simulink library "TireBody_Parameterized"  (R2026a)
settings: Solver=VariableStepAuto
undefined symbols (not defined in the file): X, Y, Z
libraries: sm_lib x4
Description:
  | Copyright 2020-2026 The MathWorks, Inc.
settings Model: Creator=smiller  LastModifiedBy=smiller

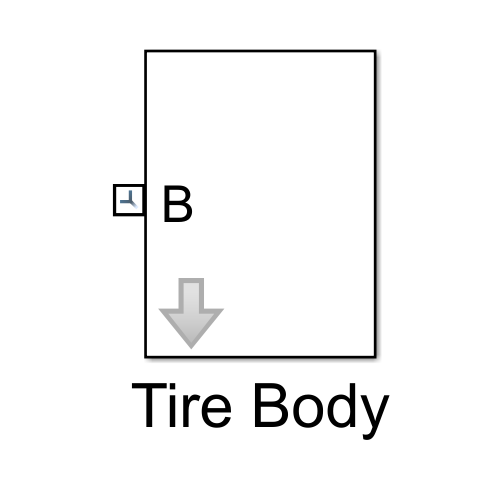
[thumbnail: Simulink's stored preview of the top-level diagram]
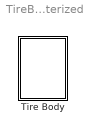
== system TireBody_Parameterized ==
  Tire Body : Subsystem  mask(Parameterized Tire Solid){radius=0.4225, rim_radius=0.3048, width=0.235, rim_width=0.235*0.1, mass=10, rim_mass=0, tire_inertia=[1 2], rim_inertia=[0 0], popup_leftRight=Left, clr_tyre=[0.5 0.5 0.5], opc_tyre=1.0, clr_rim=[0.8 0.8 0.8], opc_rim=0.5}
      mask prompts: popup_leftRight "Left/Right"
      mask help: Model mass, inertia and geometry of tire and rim.
      mask init:
      | % Change rim location if wheel is on right side
      | if (popup_leftRight == 1)
      |     rhs_tire = 1;
      | elseif(popup_leftRight == 2)
      |     rhs_tire = -1;
      | end
      | 
      | Imat = [tire_inertia(1)+rim_inertia(1) 0 0; 0 tire_inertia(1)+rim_inertia(1) 0; 0 0 tire_inertia(2)+rim_inertia(2)];
      mask TypeOptions popup_leftRight: Left | Right
      mask TypeOptions clr_tyre: Tire/GraphicDiffuseColor
      mask TypeOptions opc_tyre: Tire/GraphicOpacity
      mask TypeOptions clr_rim: Rim/GraphicDiffuseColor
      mask TypeOptions opc_rim: Rim/GraphicOpacity
      mask DialogControl cont_tyre Prompt: Tire Geometry
      mask DialogControl group_tyre_dim Prompt: Dimensions
      mask DialogControl text_tyre_tire Prompt: Tyre
      mask DialogControl text_tyre_rim Prompt: Rim
      mask DialogControl text_tyre_dim_radius Prompt: Radius (m)
      mask DialogControl text_tyre_dim_width Prompt: Width (m)
      mask DialogControl text_tyre_mass Prompt: Mass (kg)
      mask DialogControl text_tyre_inertia Prompt: Inertia [Ixx Iyy]
      mask DialogControl cont_tyre_vis Prompt: Visualization
      mask DialogControl text_vis_tyre_clr Prompt: Color [RGB]
      mask DialogControl text_vis_tyre_opc Prompt: Opacity (0-1)
      mask DialogControl text_vis_tyre_tyre Prompt: Tyre
      mask DialogControl text_vis_tyre_rim Prompt: Rim

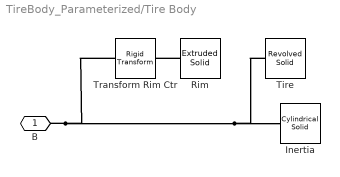
== system TireBody_Parameterized/Tire Body ==
  Inertia : sm_lib/Body Elements/Cylindrical Solid  CylinderRadius=0.001  CylinderRadiusUnits=m  CylinderLength=0.001  CylinderLengthUnits=m  ExportEntireGeometry=off  InertiaType=Custom  BasedOnType=Density  Density=1000  DensityUnits=kg/(m^3)  Mass=mass  MassUnits=kg  CenterOfMass=[0 0 0]  CenterOfMassUnits=m  MomentsOfInertia=[Imat(1,1) Imat(2,2) Imat(3,3)]  MomentsOfInertiaUnits=kg*m^2  ProductsOfInertia=[0 0 0]  ProductsOfInertiaUnits=kg*m^2  GraphicType=FromGeometry  MarkerShape=Sphere  MarkerSize=10  GraphicVisPropType=SimpleVisualProperties  GraphicDiffuseColor=[0.2 0.8 1.0]  GraphicOpacity=1.0  GraphicSpecularColor=[0.5 0.5 0.5 1.0]  GraphicAmbientColor=[0.15 0.15 0.15 1.0]  GraphicEmissiveColor=[0.0 0.0 0.0 1.0]  GraphicShininess=75  DoExposeReferenceFrame=on  SerializedFrames=<Frames/>
  Rim : sm_lib/Body Elements/Extruded Solid  ExtrusionType=Regular  PolygonNumSides=5  PolygonOuterRadius=rim_radius  PolygonOuterRadiusUnits=m  ExportEntireGeometry=off  ExtrusionCrossSection=[1 1; -1 1; -1 -1; 1 -1]  ExtrusionCrossSectionUnits=m  ExportConvexHullGeometry=off  ExtrusionLength=width*0.1  ExtrusionLengthUnits=m  InertiaType=Custom  BasedOnType=Density  Density=1000  DensityUnits=kg/(m^3)  Mass=0  MassUnits=kg  CenterOfMass=[0 0 0]  CenterOfMassUnits=m  MomentsOfInertia=[0 0 0]  MomentsOfInertiaUnits=kg*m^2  ProductsOfInertia=[0 0 0]  ProductsOfInertiaUnits=kg*m^2  GraphicType=FromGeometry  MarkerShape=Sphere  MarkerSize=10  GraphicVisPropType=SimpleVisualProperties  GraphicDiffuseColor=clr_rim  GraphicOpacity=opc_rim  GraphicSpecularColor=[0.5 0.5 0.5 1.0]  GraphicAmbientColor=[0.15 0.15 0.15 1.0]  GraphicEmissiveColor=[0.0 0.0 0.0 1.0]  GraphicShininess=75  DoExposeReferenceFrame=on  SerializedFrames=<Frames/>
  Tire : sm_lib/Body Elements/Revolved Solid  RevolutionCrossSection="[1  0.5; rim_radius/radius 0.5; rim_radius/radius -0.5; 1 -0.5].*[radius  width]"  RevolutionCrossSectionUnits=m  RevolutionExtent=Full  RevolutionAngle=180  RevolutionAngleUnits=deg  ExportConvexHullGeometry=off  InertiaType=Custom  BasedOnType=Density  Density=1000  DensityUnits=kg/(m^3)  Mass=0  MassUnits=kg  CenterOfMass=[0 0 0]  CenterOfMassUnits=m  MomentsOfInertia=[0 0 0]  MomentsOfInertiaUnits=kg*m^2  ProductsOfInertia=[0 0 0]  ProductsOfInertiaUnits=kg*m^2  GraphicType=FromGeometry  MarkerShape=Sphere  MarkerSize=10  GraphicVisPropType=SimpleVisualProperties  GraphicDiffuseColor=clr_tyre  GraphicOpacity=opc_tyre  GraphicSpecularColor=[0.5 0.5 0.5 1.0]  GraphicAmbientColor=[0.15 0.15 0.15 1.0]  GraphicEmissiveColor=[0.0 0.0 0.0 1.0]  GraphicShininess=75  DoExposeReferenceFrame=on  SerializedFrames=<Frames/>
  Transform Rim Ctr : sm_lib/Frames and Transforms/Rigid Transform  RotationMethod=None  FollAlignAxisA=+X  BaseAlignAxisA=+Y  FollAlignAxisB=+Y  BaseAlignAxisB=+Z  RotationStandardAxis=+Z  RotationAngle=0.0  RotationAngleUnits=deg  RotationArbitraryAxis=[0 0 1]  RotationSequenceAxes=FollowerAxes  RotationSequence=XYX  RotationSequenceAngles=[0 0 0]  RotationSequenceAnglesUnits=deg  RotationMatrix=[1 0 0; 0 1 0; 0 0 1]  Quaternion=[1 0 0 0]  TranslationMethod=StandardAxis  TranslationCartesianOffset=[0 0 0]  TranslationCartesianOffsetUnits=m  TranslationStandardAxis=+Z  TranslationStandardOffset=width*0.4*rhs_tire  TranslationStandardOffsetUnits=m  TranslationROffset=0  TranslationROffsetUnits=m  TranslationThetaOffset=0  TranslationThetaOffsetUnits=deg  TranslationZOffset=0  TranslationZOffsetUnits=m
  B : PMIOPort  Side=Left
  connections:
  Rim/RConn1 -- Transform Rim Ctr/RConn1
  B/RConn1 -- Transform Rim Ctr/LConn1 -- Inertia/RConn1 -- Tire/RConn1
